simulink model "PN"  (R2021a)
settings: Solver=VariableStepAuto  StartTime=0.0  StopTime=10  RelTol=1e-3
libraries: simulink_extras x1, commseqgen3 x1
settings Model: Creator=张瑞  LastModifiedBy=张瑞

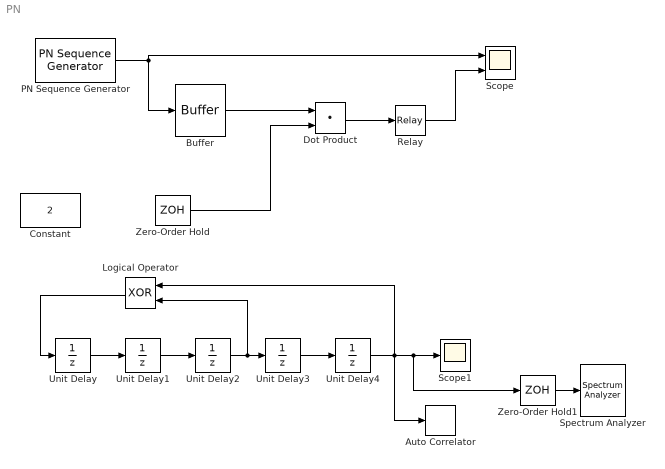
== system PN ==
  Auto Correlator : simulink_extras/Additional Sinks/Auto Correlator  npts=100  HowOften=50  sampleT=0.1
      settings: SourceProductBaseCode=SL
  Buffer : Buffer  OutputFrames=off
  Constant : Constant  Value=2  OutMin=[1]  OutMax=[5]
  Dot Product : DotProduct  InputSameDT=on  OutDataTypeStr=Inherit: Inherit via internal rule
  Logical Operator : Logic  Operator=XOR  AllPortsSameDT=off  OutDataTypeStr=boolean
  PN Sequence Generator : commseqgen3/PN Sequence Generator  poly='z^6 + z + 1'  ini_sta=[0 0 0 0 0 1]  outBitMaskSource=Dialog parameter  shift=0  outVarSiz=off  maxOutSizeMode=Dialog parameter  maxOutSize=[10 1]  Ts=1  sampPerFrame=1  reset=off  bitPackedOutputs=off  outDataType=double  numPackedBits=8  bitPackDataSigned=off  bitPackedOutDType=double
  Relay : Relay
  Scope : Scope  NumInputPorts=2
  Scope1 : Scope
  Spectrum Analyzer : SpectrumAnalyzer
  Unit Delay{,1..4} (5 alike) : UnitDelay  InitialCondition=10000  SampleTime=-1  HasFrameUpgradeWarning=on
  Zero-Order Hold : ZeroOrderHold  SampleTime=-1
  Zero-Order Hold1 : ZeroOrderHold  SampleTime=-1
  wires:
  Buffer/1 -> Dot Product/1
  PN Sequence Generator/1 -> Buffer/1, Scope/1
  Zero-Order Hold/1 -> Dot Product/2
  Dot Product/1 -> Relay/1
  Relay/1 -> Scope/2
  Unit Delay2/1 -> Logical Operator/2, Unit Delay3/1
  Unit Delay1/1 -> Unit Delay2/1
  Unit Delay/1 -> Unit Delay1/1
  Logical Operator/1 -> Unit Delay/1
  Unit Delay3/1 -> Unit Delay4/1
  Unit Delay4/1 -> Logical Operator/1, Zero-Order Hold1/1, Scope1/1, Auto Correlator/1
  Zero-Order Hold1/1 -> Spectrum Analyzer/1
